simulink model "FirstSystemsModel"  (R2024b)
settings: Solver=VariableStepAuto  StartTime=0.0  StopTime=10.0  RelTol=1e-3
values from neighbouring files (symbols this model uses):
  c = 160e-6    (= 0.00016)    [ParamTestSimulationDroop.m]    (also in ParamTestSimulatitestFirstandPI.m)
  l = 300e-6    (= 0.0003)    [ParamTestSimulationDroop.m]    (also in ParamTestSimulatitestFirstandPI.m)
  r = 0.1    [ParamTestSimulationDroop.m]    (also in ParamTestSimulatitestFirstandPI.m)
  Rc = 1e3    (= 1000)    [ParamTestSimulationDroop.m]    (also in ParamTestSimulatitestFirstandPI.m)
settings Model: Creator=rashi  LastModifiedBy=rashi

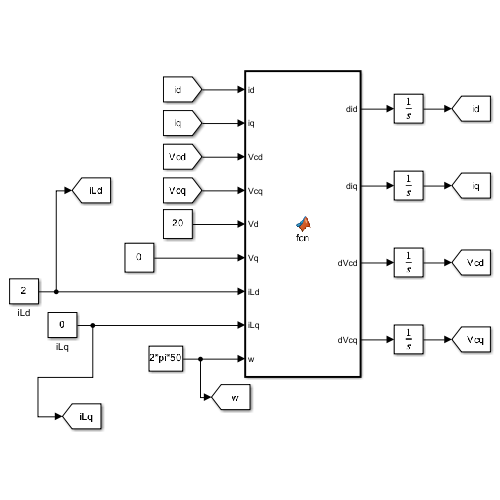
[thumbnail: Simulink's stored preview of the top-level diagram]
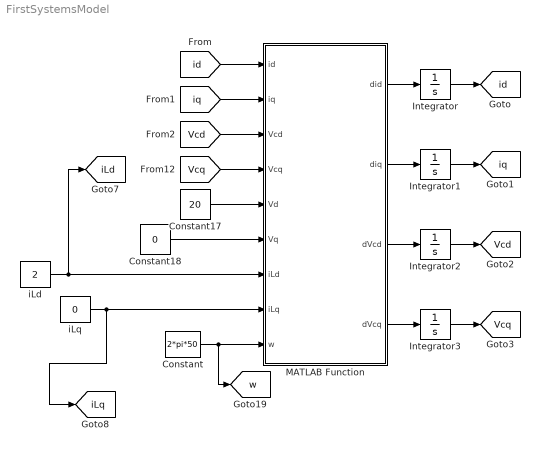
== system FirstSystemsModel ==
  Constant : Constant  Value=2*pi*50
  Constant17 : Constant  Value=20
  Constant18 : Constant  Value=0
  Integrator{,1..3} (4 alike) : Integrator
  MATLAB Function : MATLAB Function  TreatAsAtomicUnit=on
  iLd : Constant  Value=2
  iLq : Constant  Value=0
  tag scope: Vcd=global, Vcq=global, iLd=global, iLq=global, id=global, iq=global, w=global
  wires:
  Constant17/1 -> MATLAB Function/5(Vd)
  MATLAB Function/2(diq) -> Integrator1/1
  Integrator1/1 -> [iq]
  [Vcd] -> MATLAB Function/3(Vcd)
  Integrator/1 -> [id]
  MATLAB Function/1(did) -> Integrator/1
  Constant18/1 -> MATLAB Function/6(Vq)
  Integrator2/1 -> [Vcd]
  [id] -> MATLAB Function/1(id)
  Constant/1 -> [w], MATLAB Function/9(w)
  iLd/1 -> MATLAB Function/7(iLd), [iLd]
  Integrator3/1 -> [Vcq]
  iLq/1 -> [iLq], MATLAB Function/8(iLq)
  [iq] -> MATLAB Function/2(iq)
  MATLAB Function/4(dVcq) -> Integrator3/1
  [Vcq] -> MATLAB Function/4(Vcq)
  MATLAB Function/3(dVcd) -> Integrator2/1

== matlab function FirstSystemsModel/MATLAB Function ==
  data: id input; did output; iq input; Vcd input; Vcq input; Vd input; Vq input; iLd input; iLq input; w input; diq output; dVcd output; dVcq output; r parameter; l parameter; c parameter; Rc parameter
function [did,diq,dVcd,dVcq] = fcn(id,iq,Vcd,Vcq,Vd,Vq,iLd,iLq,w,r, l, c, Rc)
did = (Vd-Vcd-r*id+l*w*iq)/l;
diq = (Vq-Vcq-r*iq-l*w*id)/l;
dVcd = (id-iLd+c*w*Vcq-Vcd/Rc)/c;
dVcq = (iq-iLq-c*w*Vcd-Vcq/Rc)/c;
